simulink model "SIX_DOF_Improved"  (R2022a)
settings: Solver=FixedStepAuto  StartTime=0.0  StopTime=inf  FixedStep=1e-5  RelTol=1e-3
libraries: matrix_library x2, ros2lib x2, aerolibutil x1, aerolibanim x1, slpidlib x1
settings Model: Creator=aman  LastModifiedBy=aman

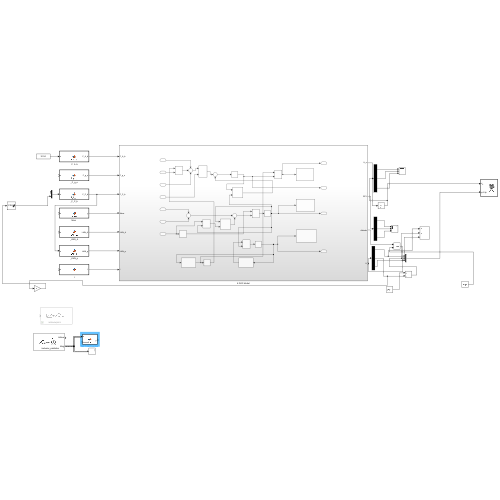
[thumbnail: Simulink's stored preview of the top-level diagram]
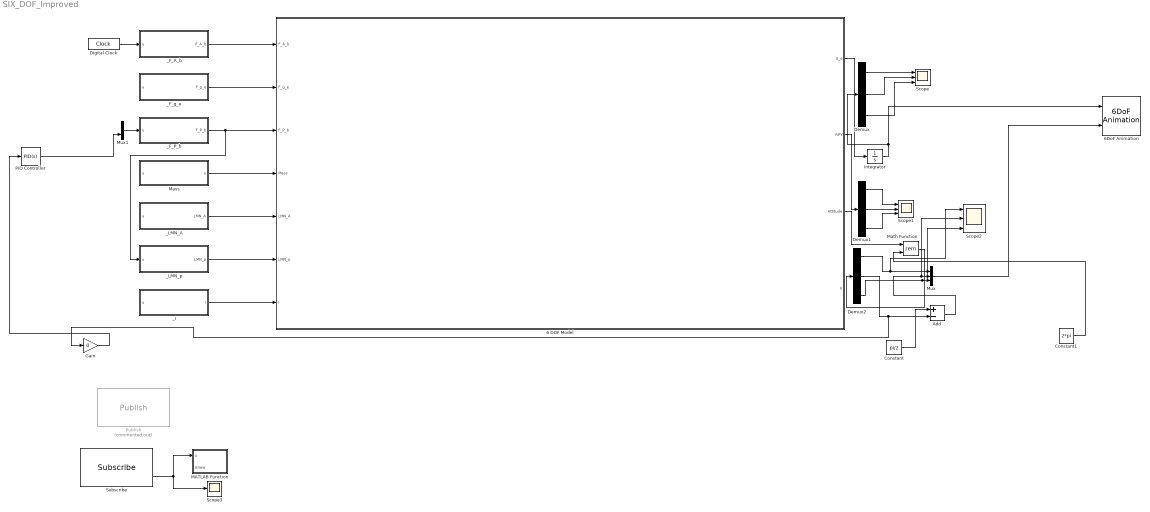
== system SIX_DOF_Improved ==
  6 DOF Model : Subsystem
  6DoF Animation : aerolibanim/6DoF Animation  u1=[0 40 -20 20 -50 -30]  u2=0.01  u3=10  u4=[4000 0 -5000]  u5=Fixed position  u6=[80 80 -126]  u7=5  u8=on
  Add : Sum  Inputs=+-
  Constant : Constant  Value=pi/2
  Constant1 : Constant  Value=2*pi
  Demux : Demux  Outputs=3
  Demux1 : Demux  Outputs=3
  Demux2 : Demux  Outputs=3
  Digital Clock : DigitalClock
  Gain : Gain  Gain=0
  Integrator : Integrator
  MATLAB Function : MATLAB Function  TreatAsAtomicUnit=on
  Mass : MATLAB Function  TreatAsAtomicUnit=on
  Math Function : Math  Operator=rem
  Mux : Mux  Inputs=3
  Mux1 : Mux  Inputs=2
  PID Controller : slpidlib/PID Controller  Controller=PID  Form=Parallel  TimeDomain=Continuous-time  UseExternalTs=off  SampleTime=-1  IntegratorMethod=Forward Euler  FilterMethod=Forward Euler  ControllerParametersSource=internal  P=8  I=0  UseKiTs=off  D=0  N=100  UseFilter=on  TunerSelectOption=Transfer Function Based (PID Tuner App)  InitialConditionSource=internal  InitialConditionForIntegrator=0  InitialConditionForFilter=0  DifferentiatorICPrevScaledInput=0  ExternalReset=none  TrackingMode=off  Kt=1  LimitOutput=on  SatLimitsSource=internal  UpperSaturationLimit=3  LowerSaturationLimit=-3  LinearizeAsGain=on  AntiWindupMode=none  Kb=1  POutMin=[]  POutMax=[]  IOutMin=[]  IOutMax=[]  DOutMin=[]  DOutMax=[]  NOutMin=[]  NOutMax=[]  SumOutMin=[]  SumOutMax=[]  SaturationOutMin=[]  SaturationOutMax=[]  PParamMin=[]  PParamMax=[]  IParamMin=[]  IParamMax=[]  DParamMin=[]  DParamMax=[]  NParamMin=[]  NParamMax=[]  KbParamMin=[]  KbParamMax=[]  KtParamMin=[]  KtParamMax=[]  KbOutMin=[]  KbOutMax=[]  KtOutMin=[]  KtOutMax=[]  IntegratorOutMin=[]  IntegratorOutMax=[]  FilterOutMin=[]  FilterOutMax=[]  SumI1OutMin=[]  SumI1OutMax=[]  SumI2OutMin=[]  SumI2OutMax=[]  SumI3OutMin=[]  SumI3OutMax=[]  SumI4OutMin=[]  SumI4OutMax=[]  SumDOutMin=[]  SumDOutMax=[]  DifferentiatorOutMin=[]  DifferentiatorOutMax=[]  FilterDiffOutCoefMin=[]  FilterDiffOutCoefMax=[]  ReciprocalOutMin=[]  ReciprocalOutMax=[]  SumDenOutMin=[]  SumDenOutMax=[]  SumNumOutMin=[]  SumNumOutMax=[]  DivideOutMin=[]  DivideOutMax=[]  UdiffTsProdOutMin=[]  UdiffTsProdOutMax=[]  NTsProdOutMin=[]  NTsProdOutMax=[]  UintegralTsProdOutMin=[]  UintegralTsProdOutMax=[]  UngainTsProdOutMin=[]  UngainTsProdOutMax=[]  IntegratorContinuousStateAttributes=''  IntegratorStateMustResolveToSignalObject=off  IntegratorRTWStateStorageClass=Auto  FilterContinuousStateAttributes=''  FilterStateMustResolveToSignalObject=off  FilterRTWStateStorageClass=Auto  ParallelPVariant=InternalParameters  IdealPVariant=Disabled  IVariant=InternalParameters  DVariant=InternalParameters  IntegratorVariant=Continuous  SatVariant=Enabled  AWVariant=Passthrough  PCopyVariant=Disabled  TRVariant=Disabled  FdbkBlocksVariant=Forward  IdealPFdbkVariant=Disabled  SatFdbkVariant=Disabled  DerivativeFilterVariant=ContFilter  NVariant=InternalParameters  NCopyVariant=Disabled  FilterICVariant=InternalICsFilter  IntegratorICVariant=InternalICs  ExternalResetVariant=Disabled  TRSumVariant=Passthrough  SumFdbkVariant=Disabled  SumVariant=Sum_PID  TsampFilterVariant=InternalTs  TsampNgainVariant=Passthrough  TsampIntegralVariant=Passthrough  ExternalSaturationOutDataTypeStr=Inherit: Same as second input  aMode=0
  Publish : ros2lib/Publish  Commented=on  topicSource=Specify your own  topic=/attitude/pitch  messageType=std_msgs/Float64  QOSHistory=Keep last  QOSDepth=1  QOSReliability=Reliable  QOSDurability=Volatile
      settings: SourceProductBaseCode=RR
  Scope : Scope  NumInputPorts=3
  Scope1 : Scope  NumInputPorts=3
  Scope2 : Scope  NumInputPorts=3
  Scope3 : Scope
  Subscribe : ros2lib/Subscribe  topicSource=Specify your own  topic=/cubemx_publisher  messageType=std_msgs/Float32  sampleTime=-1  QOSHistory=Keep last  QOSDepth=1  QOSReliability=Reliable  QOSDurability=Volatile
      settings: SourceProductBaseCode=RR
  _F_A_b : MATLAB Function  TreatAsAtomicUnit=on
  _F_P_b : MATLAB Function  TreatAsAtomicUnit=on
  _F_g_e : MATLAB Function  TreatAsAtomicUnit=on
  _I : MATLAB Function  TreatAsAtomicUnit=on
  _LMN_A : MATLAB Function  TreatAsAtomicUnit=on
  _LMN_p : MATLAB Function  TreatAsAtomicUnit=on
  wires:
  Demux1/3 -> Scope1/3
  6 DOF Model/1(U_e) -> Integrator/1
  Demux/3 -> Scope/3
  Demux/2 -> Scope/2
  Demux/1 -> Scope/1
  Demux2/3 -> Mux/3, Scope2/3
  Demux1/1 -> Scope1/1
  Mass/1(y) -> 6 DOF Model/4(Mass)
  Constant/1 -> Add/1
  Demux1/2 -> Scope1/2
  Integrator/1 -> 6DoF Animation/1, Demux/1
  _LMN_A/1(LMN_A) -> 6 DOF Model/5(LMN_A)
  Mux/1 -> 6DoF Animation/2
  Digital Clock/1 -> _F_A_b/1(u)
  Add/1 -> Scope2/2, Mux/2
  Demux2/1 -> Scope2/1, Mux/1
  _F_A_b/1(F_A_b) -> 6 DOF Model/1(F_A_b)
  _F_g_e/1(F_g_e) -> 6 DOF Model/2(F_g_e)
  _I/1(I) -> 6 DOF Model/7(I)
  _F_P_b/1(F_P_b) -> _LMN_p/1(u), 6 DOF Model/3(F_P_b)
  _LMN_p/1(LMN_p) -> 6 DOF Model/6(LMN_p)
  6 DOF Model/2(RPY) -> Demux1/1
  PID Controller/1 -> Mux1/2
  Mux1/1 -> _F_P_b/1(u)
  Demux2/2 -> Gain/1, Add/2
  6 DOF Model/3(Attitude) -> Math Function/1
  Math Function/1 -> Demux2/1
  Constant1/1 -> Math Function/2
  Gain/1 -> PID Controller/1
  Subscribe/2 -> Scope3/1, MATLAB Function/1(u)

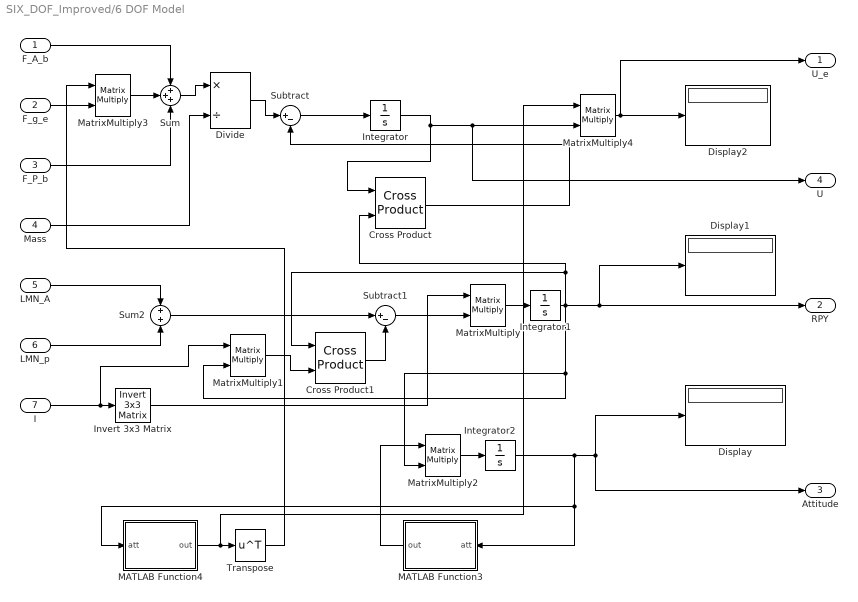
== system SIX_DOF_Improved/6 DOF Model ==
  F_A_b : Inport
  F_g_e : Inport  Port=2
  F_P_b : Inport  Port=3
  Mass : Inport  Port=4
  LMN_A : Inport  Port=5
  LMN_p : Inport  Port=6
  I : Inport  Port=7
  Cross Product : matrix_library/Cross Product
      settings: SourceProductBaseCode=SL
  Cross Product1 : matrix_library/Cross Product
      settings: SourceProductBaseCode=SL
  Display : Display
  Display1 : Display
  Display2 : Display
  Divide : Product  Inputs=*/
  Integrator : Integrator
  Integrator1 : Integrator
  Integrator2 : Integrator
  Invert 3x3 Matrix : aerolibutil/Invert  3x3 Matrix
  MATLAB Function3 : MATLAB Function  TreatAsAtomicUnit=on
  MATLAB Function4 : MATLAB Function  TreatAsAtomicUnit=on
  MatrixMultiply{,1..4} (5 alike) : Product  Multiplication=Matrix(*)
  Subtract : Sum  Inputs=|+-
  Subtract1 : Sum  Inputs=|+-
  Sum : Sum  Inputs=+++
  Sum2 : Sum  Inputs=+|+
  Transpose : Math  Operator=transpose
  U_e : Outport
  RPY : Outport  Port=2
  Attitude : Outport  Port=3
  U : Outport  Port=4
  wires:
  F_P_b/1 -> Sum/3
  F_A_b/1 -> Sum/1
  LMN_A/1 -> Sum2/1
  LMN_p/1 -> Sum2/2
  Sum/1 -> Divide/1
  Mass/1 -> Divide/2
  Divide/1 -> Subtract/1
  Subtract/1 -> Integrator/1
  Integrator/1 -> U/1, MatrixMultiply4/2, Cross Product/1
  I/1 -> MatrixMultiply1/1, Invert 3x3 Matrix/1
  Cross Product1/1 -> Subtract1/2
  Subtract1/1 -> MatrixMultiply/2
  Invert 3x3 Matrix/1 -> MatrixMultiply/1
  MatrixMultiply/1 -> Integrator1/1
  Integrator1/1 -> MatrixMultiply2/2, MatrixMultiply1/2, Display1/1, RPY/1, Cross Product/2, Cross Product1/1
  MatrixMultiply1/1 -> Cross Product1/2
  Sum2/1 -> Subtract1/1
  Cross Product/1 -> Subtract/2
  MatrixMultiply2/1 -> Integrator2/1
  Integrator2/1 -> MATLAB Function3/1(att), MATLAB Function4/1(att), Display/1, Attitude/1
  MATLAB Function3/1(out) -> MatrixMultiply2/1
  MatrixMultiply3/1 -> Sum/2
  F_g_e/1 -> MatrixMultiply3/2
  MATLAB Function4/1(out) -> MatrixMultiply4/1, Transpose/1
  Transpose/1 -> MatrixMultiply3/1
  MatrixMultiply4/1 -> Display2/1, U_e/1

== matlab function SIX_DOF_Improved/_F_A_b ==
  data: u input; F_A_b output
function F_A_b = F_A_b(u)

F_A_y_b = 0;
F_A_x_b = 0;
F_A_z_b = -12;
F_A_b = [F_A_x_b; F_A_y_b; F_A_z_b];

== matlab function SIX_DOF_Improved/_F_P_b ==
  data: u input; F_P_b output
function F_P_b = F_P_b(u)

F_P_x_b = u(2);
F_P_y_b = 0;
F_P_z_b = 0;
F_P_b = [F_P_x_b;F_P_y_b;F_P_z_b];

== matlab function SIX_DOF_Improved/Mass ==
  data: u input; y output
function y = Mass(u)

y = 1;

== matlab function SIX_DOF_Improved/_LMN_A ==
  data: u input; LMN_A output
function LMN_A = LMN_A(u)

L_A = 0.0;
M_A = 0.2;
N_A = 0;
LMN_A = [L_A;M_A;N_A];

== matlab function SIX_DOF_Improved/_I ==
  data: u input; I output
function I = I(u)

I_x = 2;
I_y = 5;
I_z = 5;
I = [I_x 0 0;0 I_y 0;0 0 I_z];

== matlab function SIX_DOF_Improved/_LMN_p ==
  data: u input; LMN_p output
function LMN_p = LMN_p(u)

N_p = 0;
L_p = u(2)*2;
M_p = u(1)*2;
LMN_p =[L_p;M_p;N_p];

== matlab function SIX_DOF_Improved/MATLAB Function ==
  data: u input; isnew input
function fcn(u,isnew)
if isnew
    disp(u.data);
end

== matlab function SIX_DOF_Improved/6 DOF Model/MATLAB Function3 ==
  data: att input size=[3 1]; out output size=[3 3]
function out = matrix(att)

out = [1 sin(att(1,1))*tan(att(2,1)) cos(att(1,1))*tan(att(2,1)) ; 0 cos(att(1,1)) -sin(att(1,1)) ; 0 sin(att(1,1))/cos(att(2,1)) cos(att(1,1))/cos(att(2,1))];

== matlab function SIX_DOF_Improved/6 DOF Model/MATLAB Function4 ==
  data: att input; out output
function out = Te_b(att)

phi = att(1,1);
theta = att(2,1);
psi = att(3,1);
out = [ cos(psi)*cos(theta)                              cos(theta)*sin(psi)                            -sin(theta); ...
         cos(psi)*sin(phi)*sin(theta)                     cos(phi)*cos(psi)+sin(phi)*sin(psi)*sin(theta) cos(theta)*sin(phi); ...
         sin(theta)*sin(psi)+cos(phi)*cos(psi)*sin(theta) cos(phi)*sin(psi)*sin(theta)-cos(psi)*sin(phi) cos(phi)*cos(theta)];

== matlab function SIX_DOF_Improved/_F_g_e ==
  data: u input; F_g_e output
function F_g_e = F_g_b(u)

F_g_x_e = 0;
F_g_y_e = 0;
F_g_z_e = 9.81;
F_g_e = [F_g_x_e;F_g_y_e;F_g_z_e];
